simulink model "hkb_coupled_osc_kelso2009"  (Simulink 10.0)
settings: Solver=ode4  StartTime=0.0  StopTime=stoptime  FixedStep=0.001  RelTol=1e-3  EnableMultiTasking=on
values from neighbouring files (symbols this model uses):
  A1 = -0.5    [run_hkb_coupled_osc_fuchs.m]
  A2 = -0.5    [run_hkb_coupled_osc_fuchs.m]
  B1 = 0.5    [run_hkb_coupled_osc_fuchs.m]
  B2 = 0.5    [run_hkb_coupled_osc_fuchs.m]
  eps1 = -8    [run_hkb_coupled_osc_fuchs.m]
  eps2 = -8    [run_hkb_coupled_osc_fuchs.m]
  eta1 = 1    [run_hkb_coupled_osc_fuchs.m]
  eta2 = 1    [run_hkb_coupled_osc_fuchs.m]
  gamma1 = 4    [run_hkb_coupled_osc_fuchs.m]
  gamma2 = 4    [run_hkb_coupled_osc_fuchs.m]
  mu2 = -1 when competitive accoridng to Kleso 2009    [run_hkb_coupled_osc_fuchs.m]
  ray1 = -0.5    [run_hkb_coupled_osc_fuchs.m]
  ray2 = -0.5    [run_hkb_coupled_osc_fuchs.m]
  wsq1 = -(omega1)^2    (= -39.4784176044)    [run_hkb_coupled_osc_fuchs.m]
  wsq2 = -(omega2)^2    (= -39.4784176044)    [run_hkb_coupled_osc_fuchs.m]
  x1_0 = 0.5    [run_hkb_coupled_osc_fuchs.m]
  x2_0 = parmat(i,1)    [run_hkb_coupled_osc_fuchs.m]
  xd1_0 = 0    [run_hkb_coupled_osc_fuchs.m]
  xd2_0 = parmat(i,2)    [run_hkb_coupled_osc_fuchs.m]
settings Model: Creator=jorda  LastModifiedBy=jorda
settings DataIOCC: SignalLoggingSaveFormat=ModelDataLogs
settings OptimizationCC: InitFltsAndDblsToZero=on
settings DebuggingCC: SaveWithParameterizedLinksMsg=none  SignalResolutionControl=TryResolveAllWithWarning  SolverPrmCheckMsg=warning  MultiTaskDSMMsg=warning  MultiTaskCondExecSysMsg=none  FcnCallInpInsideContextMsg=warning
settings SFSimCC: SimUseLocalCustomCode=on  CustomCodeUndefinedFunction=FilterOut
settings RTWCC: RTWUseLocalCustomCode=on
settings GRTTargetCC: TargetFcnLib=ansi_tfl_tmw.mat

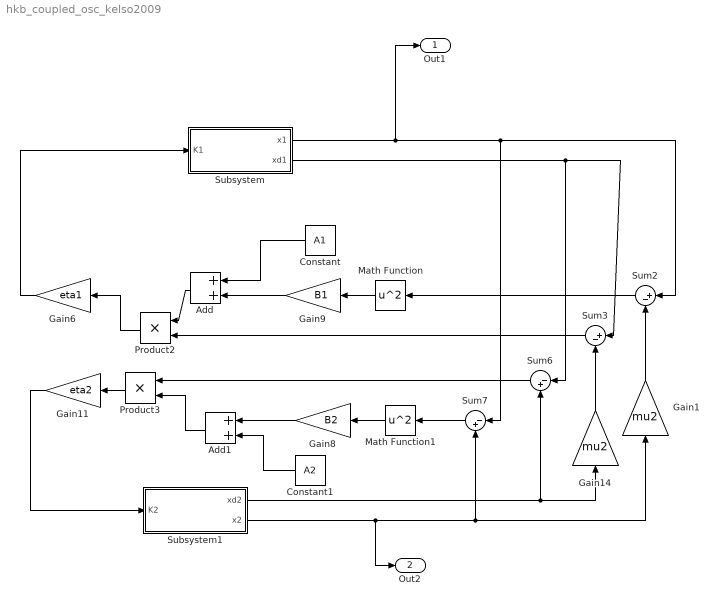
== system hkb_coupled_osc_kelso2009 ==
  Add : Sum
  Add1 : Sum
  Constant : Constant  Value=A1
  Constant1 : Constant  Value=A2
  Gain1 : Gain  Gain=mu2
  Gain11 : Gain  Gain=eta2
  Gain14 : Gain  Gain=mu2
  Gain6 : Gain  Gain=eta1
  Gain8 : Gain  Gain=B2
  Gain9 : Gain  Gain=B1
  Math Function : Math  Operator=square  SaturateOnIntegerOverflow=on
  Math Function1 : Math  Operator=square  SaturateOnIntegerOverflow=on
  Product2 : Product  RndMeth=Zero
  Product3 : Product  RndMeth=Zero
  Subsystem : Subsystem
  Subsystem1 : Subsystem
  Sum2 : Sum  Inputs=|+-
  Sum3 : Sum  Inputs=|+-
  Sum6 : Sum  Inputs=|-+
  Sum7 : Sum  Inputs=|-+
  Out1 : Outport
  Out2 : Outport  Port=2
  wires:
  Sum2/1 -> Math Function/1
  Math Function/1 -> Gain9/1
  Sum3/1 -> Product2/2
  Add/1 -> Product2/1
  Constant/1 -> Add/1
  Product2/1 -> Gain6/1
  Sum6/1 -> Product3/1
  Add1/1 -> Product3/2
  Constant1/1 -> Add1/2
  Sum7/1 -> Math Function1/1
  Math Function1/1 -> Gain8/1
  Gain8/1 -> Add1/1
  Product3/1 -> Gain11/1
  Gain9/1 -> Add/2
  Subsystem/1(x1) -> Sum2/1, Sum7/1, Out1/1
  Subsystem/2(xd1) -> Sum3/1, Sum6/1
  Gain6/1 -> Subsystem/1(K1)
  Gain11/1 -> Subsystem1/1(K2)
  Subsystem1/2(x2) -> Sum7/2, Gain1/1, Out2/1
  Subsystem1/1(xd2) -> Sum6/2, Gain14/1
  Gain14/1 -> Sum3/2
  Gain1/1 -> Sum2/2

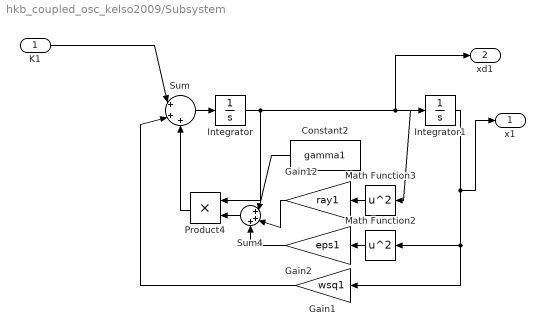
== system hkb_coupled_osc_kelso2009/Subsystem ==
  K1 : Inport
  Constant2 : Constant  Value=gamma1
  Gain1 : Gain  Gain=wsq1
  Gain12 : Gain  Gain=ray1
  Gain2 : Gain  Gain=eps1
  Integrator : Integrator  InitialCondition=xd1_0
  Integrator1 : Integrator  InitialCondition=x1_0
  Math Function2 : Math  Operator=square  SaturateOnIntegerOverflow=on
  Math Function3 : Math  Operator=square  SaturateOnIntegerOverflow=on
  Product4 : Product  RndMeth=Zero
  Sum : Sum  Inputs=|+++
  Sum4 : Sum  Inputs=|+++
  x1 : Outport
  xd1 : Outport  Port=2
  wires:
  Integrator/1 -> Product4/1, Integrator1/1, Math Function3/1, xd1/1
  Integrator1/1 -> x1/1, Gain1/1, Math Function2/1
  Sum/1 -> Integrator/1
  Math Function2/1 -> Gain2/1
  Gain1/1 -> Sum/2
  Math Function3/1 -> Gain12/1
  Constant2/1 -> Sum4/1
  Gain12/1 -> Sum4/2
  Gain2/1 -> Sum4/3
  Sum4/1 -> Product4/2
  Product4/1 -> Sum/3
  K1/1 -> Sum/1

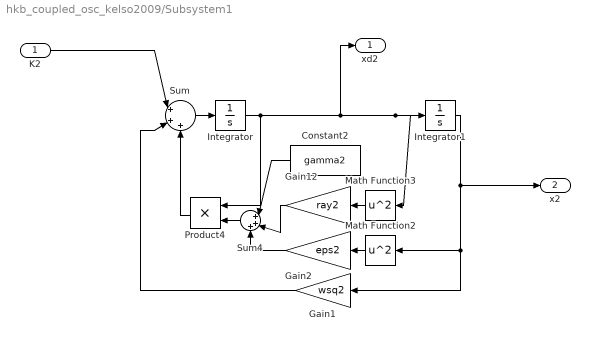
== system hkb_coupled_osc_kelso2009/Subsystem1 ==
  K2 : Inport
  Constant2 : Constant  Value=gamma2
  Gain1 : Gain  Gain=wsq2
  Gain12 : Gain  Gain=ray2
  Gain2 : Gain  Gain=eps2
  Integrator : Integrator  InitialCondition=xd2_0
  Integrator1 : Integrator  InitialCondition=x2_0
  Math Function2 : Math  Operator=square  SaturateOnIntegerOverflow=on
  Math Function3 : Math  Operator=square  SaturateOnIntegerOverflow=on
  Product4 : Product  RndMeth=Zero
  Sum : Sum  Inputs=|+++
  Sum4 : Sum  Inputs=|+++
  xd2 : Outport
  x2 : Outport  Port=2
  wires:
  Integrator/1 -> Product4/1, Integrator1/1, Math Function3/1, xd2/1
  Integrator1/1 -> Gain1/1, Math Function2/1, x2/1
  Sum/1 -> Integrator/1
  Math Function2/1 -> Gain2/1
  Gain1/1 -> Sum/2
  Math Function3/1 -> Gain12/1
  Constant2/1 -> Sum4/1
  Gain12/1 -> Sum4/2
  Gain2/1 -> Sum4/3
  Sum4/1 -> Product4/2
  Product4/1 -> Sum/3
  K2/1 -> Sum/1
